simulink model "ftbf_z"  (R2020a)
settings: Solver=VariableStepAuto  StartTime=0.0  StopTime=1  RelTol=1e-3
values from neighbouring files (symbols this model uses):
  a1 = Te/(2*ti)+t1/ti    (= 1.46428571429)    [Trottinette.m]    (also in Trottinette_couple.m = 0.707009440148)
  dCz = dCz{1}    [Trottinette.m]    (also in Trottinette_couple.m)
  dF = dF{1}    [Trottinette.m]    (also in Trottinette_2.m; Trottinette_couple.m; Trottinette_vitesse.m)
  dG = dG{1}    [Trottinette.m]    (also in Trottinette_couple.m)
  E = 0    [Trottinette.m]    (also in Trottinette_couple.m)
  I = 1/ti    (= 714.285714286)    [Trottinette.m]    (also in Trottinette_couple.m = 344.882653731)
  nCz = nCz{1}    [Trottinette.m]    (also in Trottinette_couple.m)
  nF = nF{1}    [Trottinette.m]    (also in Trottinette_2.m; Trottinette_couple.m; Trottinette_vitesse.m)
  nG = nG{1}    [Trottinette.m]    (also in Trottinette_couple.m)
  Te = 100e-6    (= 0.0001)    [Trottinette.m]    (also in Trottinette_couple.m)
libraries: simulink x1
settings Model: Creator=heusse  LastModifiedBy=heusse

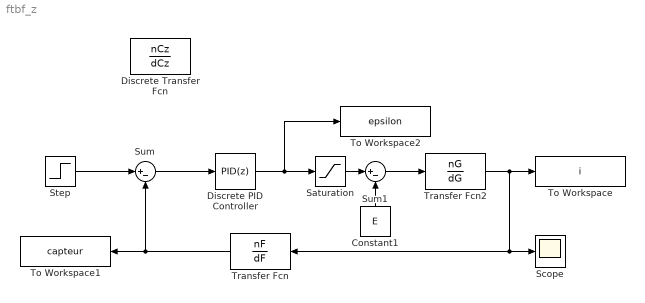
== system ftbf_z ==
  Constant1 : Constant  Value=E
  Discrete Transfer Fcn : DiscreteTransferFcn  Numerator=nCz  Denominator=dCz  SampleTime=Te
  Discrete PID Controller : simulink/Continuous/PID Controller  Controller=PID  Form=Parallel  TimeDomain=Discrete-time  UseExternalTs=off  SampleTime=Te  IntegratorMethod=Forward Euler  FilterMethod=Forward Euler  ControllerParametersSource=internal  P=a1  I=I  D=0  UseFilter=on  N=100  TunerSelectOption=Transfer Function Based (PID Tuner App)  InitialConditionSource=internal  InitialConditionForIntegrator=0  InitialConditionForFilter=0  DifferentiatorICPrevScaledInput=0  ExternalReset=none  TrackingMode=off  Kt=1  LimitOutput=on  UpperSaturationLimit=0.5  LowerSaturationLimit=-0.5  LinearizeAsGain=off  AntiWindupMode=clamping  Kb=1  POutMin=[]  POutMax=[]  IOutMin=[]  IOutMax=[]  DOutMin=[]  DOutMax=[]  NOutMin=[]  NOutMax=[]  SumOutMin=[]  SumOutMax=[]  SaturationOutMin=[]  SaturationOutMax=[]  PParamMin=[]  PParamMax=[]  IParamMin=[]  IParamMax=[]  DParamMin=[]  DParamMax=[]  NParamMin=[]  NParamMax=[]  KbParamMin=[]  KbParamMax=[]  KtParamMin=[]  KtParamMax=[]  KbOutMin=[]  KbOutMax=[]  KtOutMin=[]  KtOutMax=[]  IntegratorOutMin=[]  IntegratorOutMax=[]  FilterOutMin=[]  FilterOutMax=[]  SumI1OutMin=[]  SumI1OutMax=[]  SumI2OutMin=[]  SumI2OutMax=[]  SumI3OutMin=[]  SumI3OutMax=[]  SumI4OutMin=[]  SumI4OutMax=[]  SumDOutMin=[]  SumDOutMax=[]  DifferentiatorOutMin=[]  DifferentiatorOutMax=[]  FilterDiffOutCoefMin=[]  FilterDiffOutCoefMax=[]  ReciprocalOutMin=[]  ReciprocalOutMax=[]  SumDenOutMin=[]  SumDenOutMax=[]  SumNumOutMin=[]  SumNumOutMax=[]  DivideOutMin=[]  DivideOutMax=[]  UdiffTsProdOutMin=[]  UdiffTsProdOutMax=[]  NTsProdOutMin=[]  NTsProdOutMax=[]  UintegralTsProdOutMin=[]  UintegralTsProdOutMax=[]  UngainTsProdOutMin=[]  UngainTsProdOutMax=[]  IntegratorContinuousStateAttributes=''  IntegratorStateMustResolveToSignalObject=off  IntegratorRTWStateStorageClass=Auto  FilterContinuousStateAttributes=''  FilterStateMustResolveToSignalObject=off  FilterRTWStateStorageClass=Auto  ParallelPVariant=InternalParameters  IdealPVariant=Disabled  IVariant=InternalParameters  DVariant=InternalParameters  IntegratorVariant=Discrete  SatVariant=Enabled  AWVariant=DiscClampingParallel  PCopyVariant=Disabled  TRVariant=Disabled  FdbkBlocksVariant=Forward  IdealPFdbkVariant=Disabled  SatFdbkVariant=Disabled  DerivativeFilterVariant=ForwardEulerFilter  NVariant=InternalParameters  NCopyVariant=Disabled  FilterICVariant=InternalICsFilter  IntegratorICVariant=InternalICs  ExternalResetVariant=Disabled  TRSumVariant=Passthrough  SumFdbkVariant=Disabled  SumVariant=Sum_PID  TsampFilterVariant=InternalTs  TsampNgainVariant=Passthrough  TsampIntegralVariant=Passthrough
  Saturation : Saturate
  Scope : Scope
  Step : Step  Time=0  After=1.65  SampleTime=0
  Sum : Sum  Inputs=|+-
  Sum1 : Sum  Inputs=|+-
  To Workspace : ToWorkspace  VariableName=i  SaveFormat=Timeseries  SampleTime=-1
  To Workspace1 : ToWorkspace  VariableName=capteur  SaveFormat=Timeseries  SampleTime=-1
  To Workspace2 : ToWorkspace  VariableName=epsilon  SaveFormat=Timeseries  SampleTime=-1
  Transfer Fcn : TransferFcn  Numerator=nF  Denominator=dF
  Transfer Fcn2 : TransferFcn  Numerator=nG  Denominator=dG
  wires:
  Step/1 -> Sum/1
  Sum/1 -> Discrete PID Controller/1
  Sum1/1 -> Transfer Fcn2/1
  Discrete PID Controller/1 -> Saturation/1, To Workspace2/1
  Transfer Fcn2/1 -> To Workspace/1, Transfer Fcn/1, Scope/1
  Constant1/1 -> Sum1/2
  Saturation/1 -> Sum1/1
  Transfer Fcn/1 -> Sum/2, To Workspace1/1
